simulink model "PLANTAPRESIONLAB_CER"  (R2024a)
settings: Solver=VariableStepAuto  StartTime=0.0  StopTime=1  RelTol=1e-3
settings Model: Creator=ASUS  LastModifiedBy=ASUS

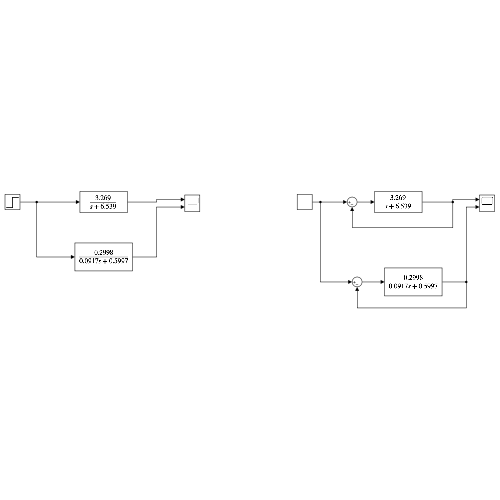
[thumbnail: Simulink's stored preview of the top-level diagram]
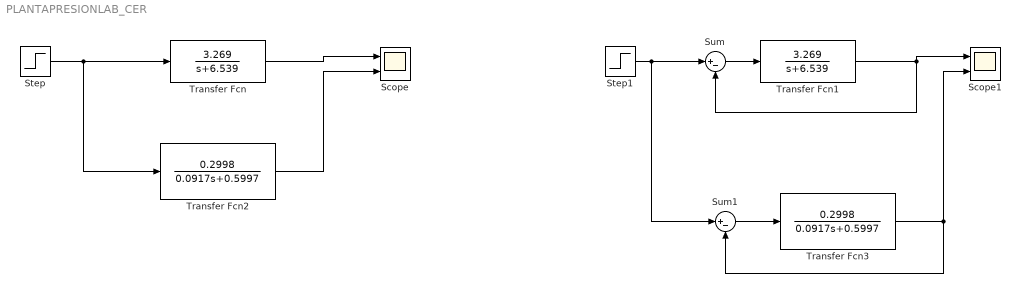
== system PLANTAPRESIONLAB_CER ==
  Scope : Scope  NumInputPorts=2
  Scope1 : Scope  NumInputPorts=2
  Step : Step  Time=0  SampleTime=0
  Step1 : Step  Time=0  After=3500  SampleTime=0
  Sum : Sum  Inputs=|+-
  Sum1 : Sum  Inputs=|+-
  Transfer Fcn : TransferFcn  Numerator=[3.269]  Denominator=[1 6.539]
  Transfer Fcn1 : TransferFcn  Numerator=[3.269]  Denominator=[1 6.539]
  Transfer Fcn2 : TransferFcn  Numerator=[0.2998]  Denominator=[0.0917 0.5997]
  Transfer Fcn3 : TransferFcn  Numerator=[0.2998]  Denominator=[0.0917 0.5997]
  wires:
  Transfer Fcn/1 -> Scope/1
  Step/1 -> Transfer Fcn2/1, Transfer Fcn/1
  Transfer Fcn1/1 -> Sum/2, Scope1/1
  Step1/1 -> Sum1/1, Sum/1
  Sum/1 -> Transfer Fcn1/1
  Transfer Fcn2/1 -> Scope/2
  Sum1/1 -> Transfer Fcn3/1
  Transfer Fcn3/1 -> Scope1/2, Sum1/2
